simulink model "Solar_Harness"  (R2025a)
settings: Solver=FixedStepAuto  StartTime=0.0  StopTime=10.0  RelTol=1e-3
libraries: fl_lib x1, nesl_utility x1, ee_lib x1
settings Model: Creator=skota  LastModifiedBy=skota
settings GRTTargetCC: UtilityFuncGeneration=Shared location

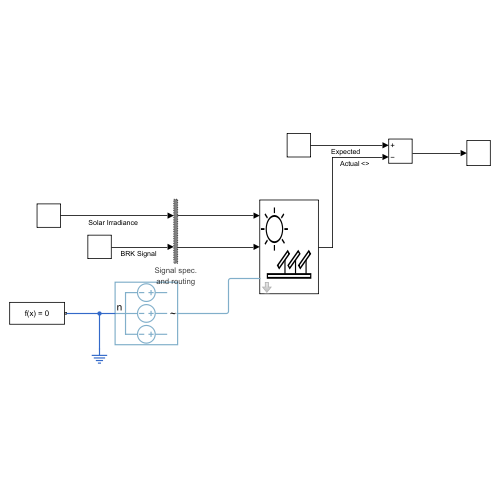
[thumbnail: Simulink's stored preview of the top-level diagram]
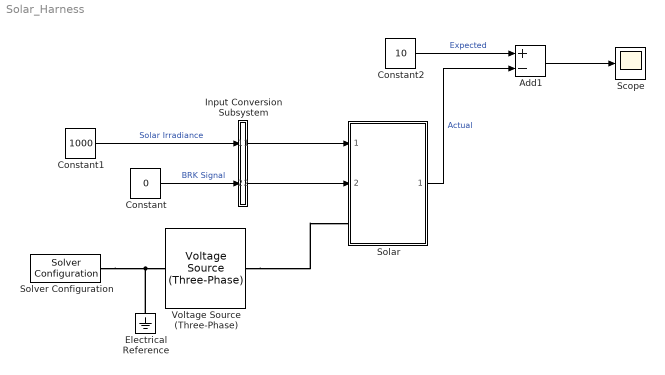
== system Solar_Harness ==
  Add1 : Sum  Inputs=+-
  Constant : Constant  Value=0
  Constant1 : Constant  Value=1000
  Constant2 : Constant  Value=10
  Electrical Reference : fl_lib/Electrical/Electrical Elements/Electrical Reference
  Input Conversion Subsystem : Subsystem  Tag=__SLT_ICS__  Description=|
      | Signal spec.
      | and routing
      settings: AttributesFormatString=%<Description>
  Scope : Scope
      settings: ActiveDisplayYMinimum=-1.22985  ActiveDisplayYMaximum=11.24887
  Solar : Subsystem  ReferencedSubsystem=Solar  maxSolarIrradiance=1000  solarRating=10  ratedVoltage=1000  Voc=37.6  panelOutput=0.25  frequency=60  windingRatio=1  MPPTVoltage="[0\t24.8912000000000\t26.3576000000000\t27.1848000000000\t27.7864000000000\t28.2376000000000\t28.5760000000000\t28.8768000000000\t29.1400000000000\t29.3656000000000\t29.5536000000000\t29.7416000000000\t29.8920000000000\t30.0424000000000\t30.1552000000000\t30.2680000000000\t30.3808000000000\t30.4560000000000\t30.5688000000000\t30.6440000000000\t30.7192000000000]"  MPPTIrradiance="[0\t50\t100\t150\t200\t250\t300\t350\t400\t450\t500\t550\t600\t650\t700\t750\t800\t850\t900\t950\t1000]"
  Solver Configuration : nesl_utility/Solver Configuration  PhysicalDomain=network_engine_domain  SubClassName=solver  LeftPortType=input  RightPortType=generic  Tones=[]  Harmonics=[]  SimulateNoise=off  Profile=off  UseLocalSampling=off  EnableSwitchedLinearOptims=on  FrequencyDomain=off  UseCCode=off  RelTol=0.001  AbsTol=0.001  MinStep=1e-09  ToWorkspace=off  RevertToSquareIcSolve=off  NumHomotopyIterations=100  PhasorMode=off  PhasorModeNumHarmonics=1  ConsistencySolver=NEWTON_XTOL_AFTER_FTOL  IndexReductionMethod=DerivativeReplacement  DoDC=off  ResidualTolerance=1e-09  ConsistencyTolSource=GLOBAL  ConsistencyAbsTol=0.001  ConsistencyRelTol=0.001  ConsistencyTolFactor=0.001  UseLocalSolver=off  LocalSolverChoice=NE_BACKWARD_EULER_ADVANCER  ResolveIndetEquations=on  FunctionEvalNumThread=1  LocalSolverSampleTime=0.001  DoFixedCost=off  MaxNonlinIter=3  MaxModeIter=2  ComputeImpulses=off  ImpulseIterations=2  LinearAlgebra=auto  LinearAlgebraNumThread=0  EquationFormulation=NE_FREQUENCY_TIME_EF  DelaysMemoryBudget=1024  AutomaticFiltering=on  FilteringTimeConstant=0.001  PartitionStorageMethod=AS_NEEDED  PartitionMemoryBudget=1024  PartitionMethod=ROBUST  MultibodyUseLocalSolver=off  MultibodyLocalSolverChoice=ODE1  MultibodyLocalSolverSampleTime=0.001
  Voltage Source (Three-Phase) : ee_lib/Sources/Voltage Source (Three-Phase)  vline_rms=1000 V  shift=0 deg  freq=60 Hz  impedance_option=0  SShortCircuit=1e6 A*V  XR=15  R=0.01 Ohm  L=3.97e-4 H  harmonic_option=0  harmonic_orders=[5, 7, 11, 13]  harmonic_ratios=[.1, .1, .1, .1]  G_parasitic=0 1/Ohm  I_specify=off  I_priority=None  I=[0, 0, 0] A  I_nominal_specify=off  I_nominal_value=1  I_nominal_unit=A
  wires:
  Solar/1 -> Add1/2  "Actual"
  Constant1/1 -> Input Conversion Subsystem/1(Inport_1)  "Solar Irradiance"
  Add1/1 -> Scope/1
  Input Conversion Subsystem/1(Outport_1) -> Solar/1
  Constant/1 -> Input Conversion Subsystem/2(Inport_2)  "BRK Signal"
  Input Conversion Subsystem/2(Outport_2) -> Solar/2
  Constant2/1 -> Add1/1  "Expected"
  connections:
  Voltage Source (Three-Phase)/RConn1 -- Solar/LConn1
  Electrical Reference/LConn1 -- Solver Configuration/RConn1 -- Voltage Source (Three-Phase)/LConn1

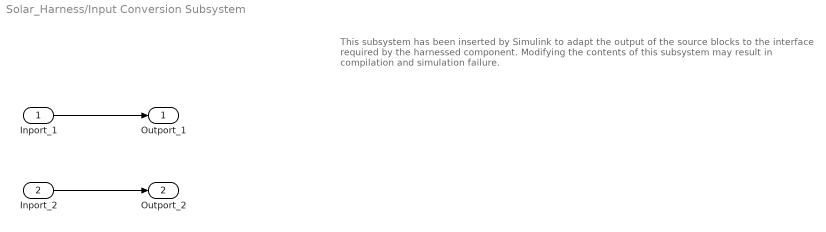
== system Solar_Harness/Input Conversion Subsystem ==
  note: This subsystem has been inserted by Simulink to adapt the output of the source blocks to the interface required by the harnessed component.
      |  Modifying the contents of this subsystem may result in compilation and simulation failure.
  Inport_1 : Inport
  Inport_2 : Inport  Port=2
  Outport_1 : Outport
  Outport_2 : Outport  Port=2
  wires:
  Inport_1/1 -> Outport_1/1
  Inport_2/1 -> Outport_2/1
